simulink model "MINI_Simscape_Assignment_03"  (R2020b)
settings: Solver=FixedStepAuto  StartTime=0.0  StopTime=10  FixedStep=0.001  MaxStep=0.01  RelTol=1e-3
InitFcn:
  | parameters;
model workspace: external: MATLAB File /Users/toricolthurst/School/ECE598IntroToHumanoid/git_humanoid/Project_Matlab/Simulation_DataFile.m (data not in the file)
values from neighbouring files (symbols this model uses):
  Butter_order = 4    [parameters.m]
  Butter_order_IMU = 8    [parameters.m]
undefined symbols (not defined in the file or in its folder): smiData, X, Y, Z
libraries: sm_lib x382, nesl_utility x115, dsparch4 x19, simulink x1
(part 8 of 8)

== matlab function MINI_Simscape_Assignment_03/MATLAB Function13 ==
  data: Left_Normal_Force input; Right_Normal_Force input; L_v input; R_v input; L_p input; R_p input; v_right_arm output; v_left_arm output; angle_right_arm output; angle_left_arm output; CLK input
function [v_right_arm, v_left_arm, angle_right_arm, angle_left_arm] = fcn(Left_Normal_Force, Right_Normal_Force, L_v, R_v, L_p, R_p, CLK)

const = 0.4;
t = 0.002;

left_foot = 0;
right_foot = 0;

if sum(Left_Normal_Force) > sum(Right_Normal_Force)
    left_foot = 1;
else
    right_foot = 1;
end

a_right_arm = 0;
a_left_arm = 0;
v_left_arm = 0;%0.2;
v_right_arm = 0;%-0.2;

inner_left = Left_Normal_Force(1) + Left_Normal_Force(3);
outer_left = Left_Normal_Force(2) + Left_Normal_Force(4);

inner_right = Right_Normal_Force(2) + Right_Normal_Force(4);
outer_right = Right_Normal_Force(1) + Right_Normal_Force(3);

if left_foot
    % stable
    if abs(inner_left - outer_left) <= .05
        a_right_arm = 0;
        a_left_arm = 0;
        v_left_arm = 0;%0.2;%0.5;
        v_right_arm = 0;%-0.2;%-0.5;
    % left arm up, right arm down
    elseif inner_left > outer_left
        a_right_arm = -1 * const * (inner_left - outer_left);   
        a_left_arm = -1 * const * (inner_left - outer_left);
        v_left_arm = -1 * const * (inner_left - outer_left);
        v_right_arm = -1.2 * const * (inner_left - outer_left);
    % right arm up, left arm down
    else
%         a_right_arm = 0;
%         a_left_arm = 0;
        a_right_arm = -1 * const * (inner_left - outer_left);
        a_left_arm = -1 * const * (inner_left - outer_left);
        v_left_arm = -1.2 * const * (inner_left - outer_left);
        v_right_arm = -1 * const * (inner_left - outer_left);
    end
elseif right_foot
    % stable
    if abs(inner_right - outer_right) <= .05
        a_right_arm = 0;
        a_left_arm = 0;
        v_left_arm = 0;%0.2;%0.5;
        v_right_arm = 0;%-0.2;%-0.5;
        % right arm up, left arm down
    elseif inner_right > outer_right
        a_right_arm = 1 * const * (inner_right - outer_right);   
        a_left_arm = 1 * const * (inner_right - outer_right);
        v_left_arm = 1.2 * const * (inner_right - outer_right);
        v_right_arm = 1 * const * (inner_right - outer_right);
    % right arm down, left arm up
    else
%         a_right_arm = 0;
%         a_left_arm = 0;
        a_right_arm = 1 * const * (inner_right - outer_right);
        a_left_arm = 1 * const * (inner_right - outer_right);
        v_left_arm = 1 * const * (inner_right - outer_right);
        v_right_arm = 1.2 * const * (inner_right - outer_right);
    end
end

% v_right_arm = R_v + a_right_arm * t;
% v_left_arm = L_v + a_left_arm * t;

% if left_foot && abs(inner_left - outer_left) <= .1
%     if L_p > -pi/4 + 0.1
%         v_left_arm = 1;
%     else
%         v_left_arm = 0;
%     end
%     if R_p > -pi/4 + 0.1
%         v_right_arm = -1;
%     else
%         v_right_arm = 0;
%     end
% end
% if right_foot && abs(inner_right - outer_right) <= .1
%     if L_p > -pi/4 + 0.1
%         v_left_arm = 1;
%     else
%         v_left_arm = 0;
%     end
%     if R_p > -pi/4 + 0.1
%         v_right_arm = -1;
%     else
%         v_right_arm = 0;
%     end
% end

angle_right_arm = R_p + v_right_arm * t %+ .5 * a_right_arm * t^2;
angle_left_arm = L_p + v_left_arm * t% + .5 * a_left_arm * t^2;

if angle_right_arm < -pi/3
    angle_right_arm = -pi/3;
elseif angle_right_arm > pi/3
    angle_right_arm = pi/3;
end

if angle_left_arm > pi/3
    angle_left_arm = pi/3;
elseif angle_left_arm < -pi/3
    angle_left_arm = -pi/3;
end

% if CLK < .01
%     v_right_arm = 0;
%     v_left_arm = 0;
%     angle_left_arm = 0;
%     angle_right_arm = 0;
% end

% if L_v == 0 && R_v == 0 && L_p == 0 && R_p == 0
%     v_right_arm = 0;
%     v_left_arm = 0;
%     angle_left_arm = 0;
%     angle_right_arm = 0;
% end

== matlab function MINI_Simscape_Assignment_03/MATLAB Function1 ==
  data: x_RH_in input; th1 output; y_RH_in input; z_RH_in input; th3 output; th5 output
% ECE 598 JK Fall 2020 University of Illinois at Urbana-Champaign
% ROBOTIS MINI Right Hand Inverse Kinematics
% 09/07/2020 by Kevin Gim (kggim2@illinois.edu)

function [th1,th3,th5] = IK_RH(x_RH_in, y_RH_in, z_RH_in)

L_sh = 39; % Origin to arm roll joint
L_a1 = 18; % Shoulder bracket horizontal distance
L_a2 = 12; % Shoulder bracket vertical distance
L_a3 = 45; % Upper arm length
L_a4 = 72; % Lower arm length

% Position of Right hand in Initial Pose (all the right arm motor angle == 0)

th1 = 0;
th3 = 0;
th5 = 0;


% Right Arm
x_RH = x_RH_in;
y_RH = y_RH_in;
z_RH = z_RH_in;
x_RH0 = x_RH;
y_RH0 = y_RH + (L_sh + L_a1);
z_RH0 = z_RH;

th1 = -atan(x_RH0/(z_RH0+0.00001))

% Range of XL320 motor -150 to 150 deg
if (th1 > 2.618)
    th1 = 2.618;
elseif (th1 < -2.618)
    th1 = -2.618;
else
    th1 = th1;
end

R1_RH = sqrt((x_RH0 - L_a2*sin(th1))^2 + y_RH0^2 + (z_RH0 + L_a2*cos(th1))^2);

if (R1_RH > 117)
    R1_RH = 117
else
    R1_RH = R1_RH;
end

alpha_RH = acos((L_a3^2 + L_a4^2 -R1_RH^2)/(2*L_a3*L_a4));

% Elbow Joint angle
th5 = -pi + alpha_RH
R2_RH = sqrt((x_RH0 - L_a2*sin(th1))^2 + (z_RH0 + L_a2*cos(th1))^2);

% Shoulder Joint angle
if (z_RH > 0)
th3 = pi/2 + (atan(y_RH0/R2_RH) + acos((L_a3^2 + R1_RH^2 - L_a4^2)/(2*L_a3*R1_RH)));
else
th3 = -pi/2 + (-atan(y_RH0/R2_RH) + acos((L_a3^2 + R1_RH^2 - L_a4^2)/(2*L_a3*R1_RH)));
end

== matlab function MINI_Simscape_Assignment_03/MATLAB Function2 ==
  data: x_LH_in input; th2 output; th4 output; th6 output; y_LH_in input; z_LH_in input
% ECE 598 JK Fall 2020 University of Illinois at Urbana-Champaign
% ROBOTIS MINI Left Hand Inverse Kinematics
% 09/07/2020 by Kevin Gim (kggim2@illinois.edu)


function [th2,th4,th6] = IK_LH(x_LH_in, y_LH_in, z_LH_in)

L_sh = 39; % Origin to arm roll joint
L_a1 = 18; % Shoulder bracket horizontal distance
L_a2 = 12; % Shoulder bracket vertical distance
L_a3 = 45; % Upper arm length
L_a4 = 72; % Lower arm length


th2 = 0;
th4 = 0;
th6 = 0;

% Left Arm
x_LH = x_LH_in;
y_LH = y_LH_in;
z_LH = z_LH_in;

x_LH0 = x_LH;
y_LH0 = y_LH - (L_sh + L_a1);
z_LH0 = z_LH;

th2 = atan(x_LH0/(z_LH0+0.00001));

% Range of XL320 motor -150 to 150 deg
if (th2 > 2.618)
    th2 = 2.618;
elseif (th2 < -2.618)
    th2 = -2.618;
else
    th2 = th2;
end

R1_LH = sqrt((x_LH0 - L_a2*sin(th2))^2 + y_LH0^2 + (z_LH0+L_a2*cos(th2))^2);

if (R1_LH > 117)
    R1_LH = 117;
else
    R1_LH = R1_LH;
end

alpha_LH = acos((L_a3^2 + L_a4^2 -R1_LH^2)/(2*L_a3*L_a4));

% Elbow Joint angle 
th6 = pi - alpha_LH;

R2_LH = sqrt((x_LH0 - L_a2*sin(th2))^2 + (z_LH0 + L_a2*cos(th2))^2);

% Shoulder Joint angle
if (z_LH0 > 0)
    th4 = -((atan(R2_LH/y_LH0) + acos((L_a3^2 + R1_LH^2 - L_a4^2)/(2*L_a3*R1_LH))));
else
    th4 = -(-pi/2 + (atan(y_LH0/R2_LH) + acos((L_a3^2 + R1_LH^2 - L_a4^2)/(2*L_a3*R1_LH))));
end

== matlab function MINI_Simscape_Assignment_03/MATLAB Function ==
  data: x_LF_in input; th8 output; y_LF_in input; z_LF_in input; roll_LF input; pitch_LF input; th10 output; th12 output; th14 output; th16 output
% ECE 598 JK Fall 2020 University of Illinois at Urbana-Champaign
% ROBOTIS MINI Left Foot Inverse Kinematics
% 09/07/2020 by Kevin Gim (kggim2@illinois.edu)

function [th8, th10, th12, th14, th16] = IK_LF(x_LF_in, y_LF_in, z_LF_in, roll_LF, pitch_LF)

%Left foot
% Controllable position x, y, z, roll, pitch

L_by = 24; % Origin to pelvis vertical length
L_bz = 72; % Pelvis horizontal length
L_bx = 15; % Shoulder joint axis to Leg center (On Sagittal Plane)
L_l1 = 6;  % Pelvis Roll axis to pitch axis
L_l2 = 45; % Thigh Length
L_l3 = 42; % Shank Length
L_l4 = 31;  % Ankle Length
L_f = 9; % Foot horizontal length

x_LF = x_LF_in;
y_LF = y_LF_in;
z_LF = z_LF_in;


R0LF = RX(roll_LF) * RY(pitch_LF);
T0LF = R0LF + TXYZ(x_LF, y_LF, z_LF) - eye(4);
T016 = T0LF * RY(-(pi)/2) *RZ((pi)) * TXYZ(-L_l4,L_f,0);
TLF0_16 = inv(TXYZ(L_bx,L_by,-L_bz)*RY((pi)/2))*T016;
pos_LF = TLF0_16(1:3,4);

th8 = atan(pos_LF(2)/pos_LF(1))
R1_LF = sqrt((pos_LF(1)-L_l1*cos(th8))^2 + (pos_LF(2)-L_l1*sin(th8))^2 + pos_LF(3)^2);
alpha_LF = acos((L_l2^2 + L_l3^2 -R1_LF^2)/(2*L_l2*L_l3));

th12 = -pi+alpha_LF
R2_LF = sqrt((pos_LF(1)-L_l1*cos(th8))^2 + (pos_LF(2)-L_l1*sin(th8))^2);

th10 = (atan(pos_LF(3)/R2_LF) + acos((L_l2^2 + R1_LF^2 - L_l3^2)/(2*L_l2*R1_LF)));


T_LF0_12 = [ cos(th10 + th12)*cos(th8), -sin(th10 + th12)*cos(th8),  sin(th8), cos(th8)*(L_l1 + L_l2*cos(th10));
    cos(th10 + th12)*sin(th8), -sin(th10 + th12)*sin(th8), -cos(th8), sin(th8)*(L_l1 + L_l2*cos(th10));
    sin(th10 + th12),           cos(th10 + th12),         0,                   L_l2*sin(th10);
    0,                          0,         0,                                1]

T_12_16 = inv(T_LF0_12)*TLF0_16;
th14 = -acos(-T_12_16(2,3));
th16 = asin(-T_12_16(3,1));

== matlab function MINI_Simscape_Assignment_03/MATLAB Function3 ==
  data: x_RF_in input; th7 output; y_RF_in input; z_RF_in input; roll_RF input; pitch_RF input; th9 output; th11 output; th13 output; th15 output
% ECE 598 JK Fall 2020 University of Illinois at Urbana-Champaign
% ROBOTIS MINI Right Foot Inverse Kinematics
% 09/07/2020 by Kevin Gim (kggim2@illinois.edu)

function [th7,th9, th11, th13, th15] = IK_RF(x_RF_in, y_RF_in, z_RF_in, roll_RF, pitch_RF)

% Right foot
% Controllable position x, y, z, roll, pitch

L_by = 24; % Origin to pelvis vertical length
L_bz = 72; % Pelvis horizontal length
L_bx = 15; % Shoulder joint axis to Leg center (On Sagittal Plane)
L_l1 = 6;  % Pelvis Roll axis to pitch axis
L_l2 = 45; % Thigh Length
L_l3 = 42; % Shank Length
L_l4 = 31;  % Ankle Length
L_f = 9; % Foot horizontal length

x_RF = x_RF_in;
y_RF = y_RF_in;
z_RF = z_RF_in;

R0RF = RX(roll_RF) * RY(pitch_RF);
T0RF = R0RF + TXYZ(x_RF, y_RF, z_RF) - eye(4);
T015 = T0RF * RY(-(pi)/2) * RZ((pi)) * TXYZ(-L_l4,-L_f,0);
TRF0_15 = inv(TXYZ(L_bx,-L_by,-L_bz)*RY((pi)/2))*T015;

pos_RF = TRF0_15(1:3,4);
th7 = atan(pos_RF(2)/pos_RF(1));
R1_RF = sqrt((pos_RF(1)-L_l1*cos(th7))^2 + (pos_RF(2)-L_l1*sin(th7))^2 + pos_RF(3)^2);
alpha_RF = acos((L_l2^2 + L_l3^2 -R1_RF^2)/(2*L_l2*L_l3));
th11 = pi-alpha_RF;
R2_RF = sqrt((pos_RF(1)-L_l1*cos(th7))^2 + (pos_RF(2)-L_l1*sin(th7))^2);

th9 = -((atan(pos_RF(3)/R2_RF) + acos((L_l2^2 + R1_RF^2 - L_l3^2)/(2*L_l2*R1_RF))));

T_RF0_11 = [ cos(th9 + th11)*cos(th7), -sin(th9 + th11)*cos(th7), -sin(th7), cos(th7)*(L_l1 + L_l2*cos(th9));
    cos(th9 + th11)*sin(th7), -sin(th9 + th11)*sin(th7),  cos(th7), sin(th7)*(L_l1 + L_l2*cos(th9));
    -sin(th9 + th11),          -cos(th9 + th11),         0,                  -L_l2*sin(th9);
    0,                         0,         0,                               1];

T_11_15 = inv(T_RF0_11)*TRF0_15;
th13 = asin(T_11_15(1,3));
th15 = -asin(-T_11_15(3,1));

== matlab function MINI_Simscape_Assignment_03/MATLAB Function4 ==
  data: P_CoM_wholebody output; joint_angle input; P_CoM_part output
function [P_CoM_wholebody, P_CoM_part] = COM_FK(joint_angle)

% CoM Calculation code
% Input: joint Angles
% Output: 1) P_CoM_part: 3 x 17 matrix of CoM positions of each links. Each
%            column contains CoM position of each links with respect to the 
%            frame 0. [CoM_x; CoM_y; CoM_z;]
%
%         2) P_CoM_wholebody: 3x1 array of the position of the whole body
%            CoM [CoM_x; CoM_y; CoM_z;]

coder.extrinsic('-sync:on','DHparameter');
coder.extrinsic('-sync:on','TXYZ');
coder.extrinsic('-sync:on','RX');
coder.extrinsic('-sync:on','RY');
coder.extrinsic('-sync:on','RZ');

th1 = joint_angle(1); th3 = joint_angle(2); th5 = joint_angle(3);
th2 = joint_angle(4); th4 = joint_angle(5); th6 = joint_angle(6);
th7 = joint_angle(7); th9 = joint_angle(8); th11 = joint_angle(9); th13 = joint_angle(10); th15 = joint_angle(11);
th8 = joint_angle(12); th10 = joint_angle(13); th12 = joint_angle(14); th14 = joint_angle(15); th16 =joint_angle(16);

L_sh = 39; % Origin to arm roll joint
L_a1 = 18; % Shoulder bracket horizontal distance
L_a2 = 12; % Shoulder bracket vertical distance
L_a3 = 45; % Upper arm length
L_a4 = 72; % Lower arm length

L_by = 24; % Origin to pelvis vertical length
L_bz = 72; % Pelvis horizontal length
L_bx = 15; % Shoulder joint axis to Leg center (On Sagittal Plane)
L_l1 = 6;  % Pelvis Roll axis to pitch axis
L_l2 = 45; % Thigh Length
L_l3 = 42; % Shank Length
L_l4 = 31;  % Ankle Length


m_body = 250.48;
m_arm1 = 4.26;
m_arm2 = 23;
m_arm3 = 26.16;
m_leg1 = 19.9;
m_leg2 = 23;
m_leg3 = 8.99;
m_leg4 = 19.57;
m_leg5 = 36.53;

T_RH = zeros(4,4,4);
T_LH = zeros(4,4,4);
T_RF = zeros(4,4,6);
T_LF = zeros(4,4,6);

T_RH_all = zeros(4,4,4);
T_LH_all = zeros(4,4,4);
T_RF_all = zeros(4,4,6);
T_LF_all = zeros(4,4,6);

P_CoM_part_temp = zeros(4,17);
P_CoM_part = zeros(3,17)

% CoM Location
CoM_body = [-1.77; 0; -21.33];
CoM_RH_1 = [4.57; 0; -8.85];
CoM_RH_2 = [12.05; 0.97; -0.05];
CoM_RH_3 = [20; 1.29; 0.18];
CoM_LH_1 = [4.57; 0; -8.85];
CoM_LH_2 = [12.05; -0.97; -0.05];
CoM_LH_3 = [20; -1.29; 0.18];
CoM_RF_1 = [-1.22; -0.06; -1.47];
CoM_RF_2 = [32.95; -0.97; -0.05];
CoM_RF_3 = [17.90; -6.88; 0];
CoM_RF_4 = [-6.23; -1.76; 0.06];
CoM_RF_5 = [12.25; 8.01; 21.06];
CoM_LF_1 = [-1.22; 0.06; -1.47];
CoM_LF_2 = [32.95; 0.97; -0.05];
CoM_LF_3 = [17.90; 6.88; 0];
CoM_LF_4 = [-6.23; 1.76; 0.06];
CoM_LF_5 = [12.25; -8.01; 21.06];

% Right Hand
% DH parameter starts from arm origin at the shoulder
%    [a   alpha  d  theta]
DH_RH = [0, 0, 0, th1-(pi)/2;
    L_a2, (pi)/2, 0, (pi)/2+th3;
    L_a3, 0, 0, th5;
    L_a4, 0, 0, 0];

T_RH_all = DHparameter(DH_RH);
T_RH(:,:,1) = TXYZ(0,-(L_sh+L_a1),0)*RX((pi)/2)*T_RH_all(:,:,1);
T_RH(:,:,2) = T_RH(:,:,1)*T_RH_all(:,:,2);
T_RH(:,:,3) = T_RH(:,:,2)*T_RH_all(:,:,3);
T_RH(:,:,4) = T_RH(:,:,3)*T_RH_all(:,:,4);

P_CoM_part_temp(:,1) = T_RH(:,:,1)*[CoM_RH_1;1];
P_CoM_part_temp(:,2) = T_RH(:,:,2)*[CoM_RH_2;1];
P_CoM_part_temp(:,3) = T_RH(:,:,3)*[CoM_RH_3;1];

% Left Hand
% DH parameter starts from arm origin at the shoulder
% Modified DH
%    [a   alpha  d  theta]
DH_LH = [0, 0, 0, th2+(pi)/2;
    L_a2, -(pi)/2, 0, -(pi)/2+th4;
    L_a3, 0, 0, th6;
    L_a4, 0, 0, 0];

T_LH_all = DHparameter(DH_LH);
T_LH(:,:,1) = TXYZ(0,L_sh+L_a1,0)*RX(-(pi)/2)*T_LH_all(:,:,1);
T_LH(:,:,2) = T_LH(:,:,1)*T_LH_all(:,:,2);
T_LH(:,:,3) = T_LH(:,:,2)*T_LH_all(:,:,3);
T_LH(:,:,4) = T_LH(:,:,3)*T_LH_all(:,:,4);

P_CoM_part_temp(:,4) = T_LH(:,:,1)*[CoM_LH_1;1];
P_CoM_part_temp(:,5) = T_LH(:,:,2)*[CoM_LH_2;1];
P_CoM_part_temp(:,6) = T_LH(:,:,3)*[CoM_LH_3;1];


% Right Foot
% DH parameter starts from the hip roll joint
%    [a   alpha  d  theta]
DH_RF = [0, 0, 0, th7;
    L_l1,-(pi)/2, 0, th9;
    L_l2, 0, 0, th11;
    L_l3, pi, 0, th13;
    0, pi/2, 0, th15;
    L_l4, 0, 0, 0];

T_RF_all = DHparameter(DH_RF);
T_RF(:,:,1) = TXYZ(L_bx,-L_by,-L_bz)*RY((pi)/2)*T_RF_all(:,:,1);
T_RF(:,:,2) = T_RF(:,:,1)*T_RF_all(:,:,2);
T_RF(:,:,3) = T_RF(:,:,2)*T_RF_all(:,:,3);
T_RF(:,:,4) = T_RF(:,:,3)*T_RF_all(:,:,4);
T_RF(:,:,5) = T_RF(:,:,4)*T_RF_all(:,:,5);
T_RF(:,:,6) = T_RF(:,:,5)*T_RF_all(:,:,6);

P_CoM_part_temp(:,7) = T_RF(:,:,1)*[CoM_RF_1;1];
P_CoM_part_temp(:,8) = T_RF(:,:,2)*[CoM_RF_2;1];
P_CoM_part_temp(:,9) = T_RF(:,:,3)*[CoM_RF_3;1];
P_CoM_part_temp(:,10) = T_RF(:,:,4)*[CoM_RF_4;1];
P_CoM_part_temp(:,11) = T_RF(:,:,5)*[CoM_RF_5;1];

% Left Foot
% DH parameter starts from the hip roll joint
%    [a   alpha  d  theta]
DH_LF = [0, 0, 0, th8;
    L_l1,(pi)/2, 0, th10;
    L_l2, 0, 0, th12;
    L_l3, pi, 0, th14;
    0, -pi/2, 0, th16
    L_l4, 0, 0, 0];

T_LF_all = DHparameter(DH_LF);
T_LF(:,:,1) = TXYZ(L_bx,L_by,-L_bz)*RY((pi)/2)*T_LF_all(:,:,1);
T_LF(:,:,2) = T_LF(:,:,1)*T_LF_all(:,:,2);
T_LF(:,:,3) = T_LF(:,:,2)*T_LF_all(:,:,3);
T_LF(:,:,4) = T_LF(:,:,3)*T_LF_all(:,:,4);
T_LF(:,:,5) = T_LF(:,:,4)*T_LF_all(:,:,5);
T_LF(:,:,6) = T_LF(:,:,5)*T_LF_all(:,:,6);

P_CoM_part_temp(:,12) = T_LF(:,:,1)*[CoM_LF_1;1];
P_CoM_part_temp(:,13) = T_LF(:,:,2)*[CoM_LF_2;1];
P_CoM_part_temp(:,14) = T_LF(:,:,3)*[CoM_LF_3;1];
P_CoM_part_temp(:,15) = T_LF(:,:,4)*[CoM_LF_4;1];
P_CoM_part_temp(:,16) = T_LF(:,:,5)*[CoM_LF_5;1];
P_CoM_part_temp(:,17) = [CoM_body;1];
%% Calculate Wholebody COM

P_CoM_wholebody = (P_CoM_part_temp(1:3,17)*m_body ...
    + P_CoM_part_temp(1:3,1)*m_arm1 + P_CoM_part_temp(1:3,2)*m_arm2 + P_CoM_part_temp(1:3,3)*m_arm3 ...
    + P_CoM_part_temp(1:3,4)*m_arm1 + P_CoM_part_temp(1:3,5)*m_arm2 + P_CoM_part_temp(1:3,6)*m_arm3 ...
    + P_CoM_part_temp(1:3,7)*m_leg1 + P_CoM_part_temp(1:3,8)*m_leg2 + P_CoM_part_temp(1:3,9)*m_leg3 + P_CoM_part_temp(1:3,10)*m_leg4 + P_CoM_part_temp(1:3,11)*m_leg5 ...
    + P_CoM_part_temp(1:3,12)*m_leg1 + P_CoM_part_temp(1:3,13)*m_leg2 + P_CoM_part_temp(1:3,14)*m_leg3 + P_CoM_part_temp(1:3,15)*m_leg4 + P_CoM_part_temp(1:3,16)*m_leg5)...
    /(m_body + 2*(m_arm1 + m_arm2 + m_arm3)+ 2*(m_leg1 + m_leg2 + m_leg3 + m_leg4 + m_leg5));

P_CoM_part = P_CoM_part_temp(1:3,:);

== matlab function MINI_Simscape_Assignment_03/MATLAB Function5 ==
  data: Left_Friction_Sensor input; Left_Slip output; Left_Normal_Force input; Right_Friction_Sensor input; Right_Normal_Force input; L_vx input; L_vy input; R_vx input; R_vy input; Right_Slip output
function [Left_Slip, Right_Slip] = slip_prediction(Left_Friction_Sensor, Left_Normal_Force, Right_Friction_Sensor, Right_Normal_Force, L_vx, L_vy, R_vx, R_vy)

mu = .6;
V_critical = 1e-2;

Left_Slip = zeros(1, 4);
Right_Slip = zeros(1, 4);

for i = 1:4
    if sqrt(L_vx(i)^2 + L_vy(i)^2) > V_critical
        mu = .1;
    else
        mu = .02;
    end

    Left_Slip(i) = Left_Normal_Force(i) * mu;
    
    if sqrt(R_vx(i)^2 + R_vy(i)^2) > V_critical
        mu = .1;
    else
        mu = .02;
    end
    Right_Slip(i) = Right_Normal_Force(i) * mu;
end
